simulink model "verify_Valve_ThermoTset_mdl"  (R2016b)
settings: Solver=ode45  StartTime=0.0  StopTime=600  MaxStep=1  RelTol=1e-3  EnableMultiTasking=on
libraries: carnot x3
settings Model: Creator=drhf  LastModifiedBy=srrt
settings DataIOCC: SaveFormat=Array  SignalLoggingSaveFormat=ModelDataLogs
settings OptimizationCC: ExpressionDepthLimit=2147483647  LifeSpan=inf
settings DebuggingCC: UnderspecifiedInitializationDetection=Classic  MergeDetectMultiDrivingBlocksExec=none  SolverPrmCheckMsg=warning  FcnCallInpInsideContextMsg=warning  StateNameClashWarn=warning  SFUnexpectedBacktrackingDiag=warning  SFNoUnconditionalDefaultTransitionDiag=warning  SFExecutionAtInitializationDiag=none
settings HardwareCC: ProdBitPerPointer=32  ProdBitPerSizeT=32  ProdBitPerPtrDiffT=32  ProdLargestAtomicFloat=None  ProdIntDivRoundTo=Undefined  ProdEndianess=Unspecified  ProdWordSize=32  ProdHWDeviceType=32-bit Generic
settings ModelReferenceCC: PropagateSignalLabelsOutOfModel=off
settings GRTTargetCC: TargetLangStandard=C89/C90 (ANSI)  GeneratePreprocessorConditionals=Disable all  CombineOutputUpdateFcns=off  GRTInterface=on
settings ConfigComp: CovMetricSettings=dw  CovHtmlReporting=on  CovSaveCumulativeToWorkspaceVar=on  CovSaveSingleToWorkspaceVar=on  CovExternalEMLEnable=off

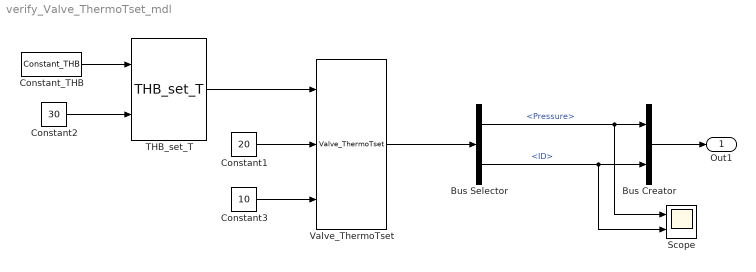
== system verify_Valve_ThermoTset_mdl ==
  Bus Creator : BusCreator  Inputs=2
  Bus Selector : BusSelector  OutputSignals=Pressure,ID
  Constant1 : Constant  Value=20
  Constant2 : Constant  Value=30
  Constant3 : Constant  Value=10
  Constant_THB : carnot/Source/Simple/Constant_THB  t=40  mdot=720/3600  p=1e5  mID=No Pressure Drop  fluid=Water  mix=0  mix2=0  mix3=0  dia=10  hgt=0
  Scope : Scope  NumInputPorts=2
  THB_set_T : carnot/Source/Simple/THB_set_T
  Valve_ThermoTset : carnot/Hydraulics/Valve_ThermoTset  p=3  op=0.5  bl=10  ts=30  dia=0.02  vpos=[0 0.1 1]  vqua=[1e6 1e6 1]
  Out1 : Outport
  wires:
  Bus Creator/1 -> Out1/1
  Bus Selector/1 -> Scope/1, Bus Creator/1  "<Pressure>"
  Bus Selector/2 -> Scope/2, Bus Creator/2  "<ID>"
  Valve_ThermoTset/1 -> Bus Selector/1
  Constant1/1 -> Valve_ThermoTset/2
  Constant_THB/1 -> THB_set_T/1
  THB_set_T/1 -> Valve_ThermoTset/1
  Constant2/1 -> THB_set_T/2
  Constant3/1 -> Valve_ThermoTset/3
